simulink model "helicopter_hat"  (R2024a)
settings: Solver=VariableStepAuto  StartTime=0.0  StopTime=T  RelTol=1e-4
undefined symbols (not defined in the file or in its folder): b, K1, K3, K4
settings Model: Creator=lcaric  LastModifiedBy=piotr
settings SolverCC: AlgebraicLoopSolver=TrustRegion
settings DataIOCC: ReturnWorkspaceOutputs=off
settings DebuggingCC: UnconnectedInputMsg=warning  UnconnectedOutputMsg=warning  UnconnectedLineMsg=warning  ArithmeticOperatorsInVariantConditions=warning
settings ModelReferenceCC: EnableRefExpFcnMdlSchedulingChecks=on
settings SFSimCC: CustomCodeUndefinedFunction=UseInterfaceOnly
settings RTWCC: GPUComputeCapability=3.5

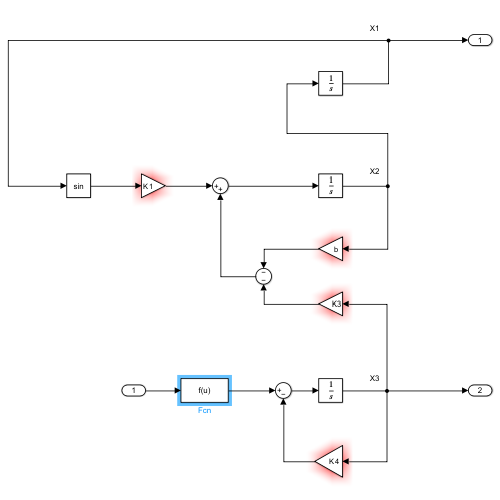
[thumbnail: Simulink's stored preview of the top-level diagram]
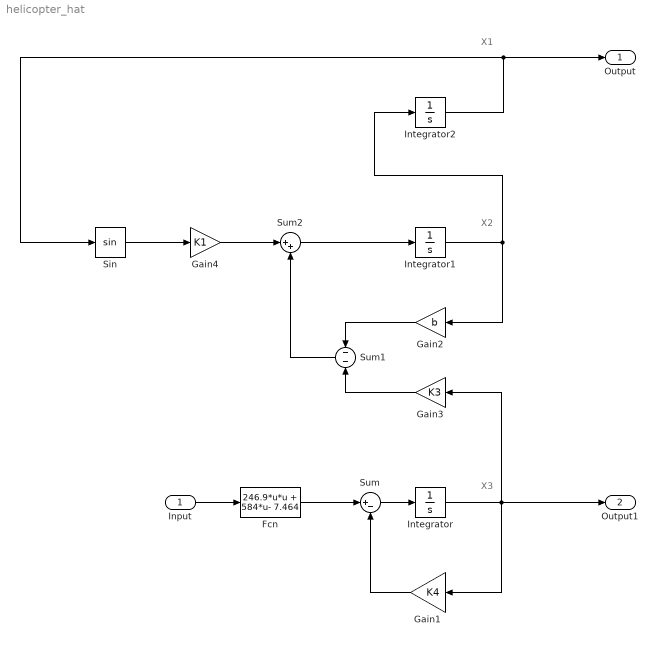
== system helicopter_hat ==
  note: X1
  note: X2
  note: X3
  Input : Inport
  Fcn : Fcn  Expr=246.9*u*u + 584*u- 7.464
  Gain1 : Gain  Gain=K4
  Gain2 : Gain  Gain=b
  Gain3 : Gain  Gain=K3
  Gain4 : Gain  Gain=K1
  Integrator : Integrator
  Integrator1 : Integrator
  Integrator2 : Integrator
  Sin : Trigonometry
  Sum : Sum  Inputs=|+-
  Sum1 : Sum  Inputs=--
  Sum2 : Sum  Inputs=|++
  Output : Outport  VectorParamsAs1DForOutWhenUnconnected=off
  Output1 : Outport  Port=2  VectorParamsAs1DForOutWhenUnconnected=off
  wires:
  Fcn/1 -> Sum/1
  Gain1/1 -> Sum/2
  Sum/1 -> Integrator/1
  Integrator/1 -> Gain1/1, Output1/1, Gain3/1
  Gain2/1 -> Sum1/1
  Gain3/1 -> Sum1/2
  Integrator1/1 -> Gain2/1, Integrator2/1
  Integrator2/1 -> Output/1, Sin/1
  Sum1/1 -> Sum2/2
  Sin/1 -> Gain4/1
  Sum2/1 -> Integrator1/1
  Gain4/1 -> Sum2/1
  Input/1 -> Fcn/1
